simulink model "pipeline_12bit_not_ideal"  (R2017b)
settings: Solver=FixedStepAuto  StartTime=0.0  StopTime=5000*ts  FixedStep=ts  RelTol=1e-3
values from neighbouring files (symbols this model uses):
  bits_number = 12    [launch_pipeline_12ibt.m]
  fin = antismear(fin_pre,fs,nfft)    [launch_pipeline_12ibt.m]
  ts = 1/fs    (= 1)    [launch_pipeline_12ibt.m]
undefined symbols (not defined in the file or in its folder): clock
libraries: SDtoolbox x8
settings Model: Creator=umi  LastModifiedBy=SHUOGE
settings DataIOCC: LimitDataPoints=on  SaveFormat=Array  SaveOutput=off  SaveTime=off
settings OptimizationCC: ExpressionDepthLimit=2147483647  LifeSpan=inf
settings DebuggingCC: UnderspecifiedInitializationDetection=Classic  MergeDetectMultiDrivingBlocksExec=none  SolverPrmCheckMsg=warning  StateNameClashWarn=warning  SFUnexpectedBacktrackingDiag=warning  SFNoUnconditionalDefaultTransitionDiag=warning  SFExecutionAtInitializationDiag=none
settings HardwareCC: ProdBitPerPointer=32  ProdBitPerSizeT=32  ProdBitPerPtrDiffT=32  ProdLargestAtomicFloat=None  ProdIntDivRoundTo=Undefined  ProdEndianess=Unspecified  ProdWordSize=32  ProdHWDeviceType=32-bit Generic
settings ModelReferenceCC: PropagateSignalLabelsOutOfModel=off
settings CodeAppCC: StateflowObjectComments=on
settings GRTTargetCC: TargetLangStandard=C89/C90 (ANSI)  GeneratePreprocessorConditionals=Disable all  CombineOutputUpdateFcns=off  GRTInterface=on
settings ConfigComp: CovMetricSettings=dw  CovHtmlReporting=on  CovSaveCumulativeToWorkspaceVar=on  CovSaveSingleToWorkspaceVar=on  CovExternalEMLEnable=off  CovSFcnEnable=off

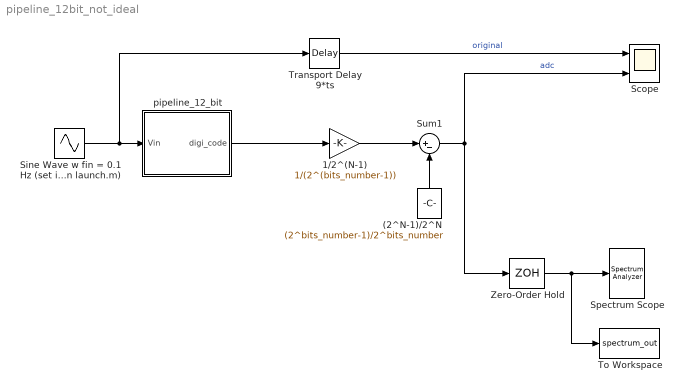
== system pipeline_12bit_not_ideal ==
  (2^N-1)/2^N : Constant  Value=(2^bits_number-1)/2^bits_number
  1/2^(N-1) : Gain  Gain=1/(2^(bits_number-1))
  Scope : Scope  NumInputPorts=2
  Sine Wave w fin = 0.1 Hz (set in launch.m) : Sin  Frequency=2*pi*fin  SampleTime=0
  Spectrum Scope : SpectrumAnalyzer
  Sum1 : Sum  Inputs=|+-
  To Workspace : ToWorkspace  VariableName=spectrum_out  SampleTime=-1
  Transport Delay 9*ts : TransportDelay  DelayTime=9
  Zero-Order Hold : ZeroOrderHold
  pipeline_12_bit : Subsystem
  wires:
  Sum1/1 -> Scope/2, Zero-Order Hold/1  "adc"
  (2^N-1)/2^N/1 -> Sum1/2
  1/2^(N-1)/1 -> Sum1/1
  pipeline_12_bit/1(digi_code) -> 1/2^(N-1)/1
  Sine Wave w fin = 0.1 Hz (set in launch.m)/1 -> pipeline_12_bit/1(Vin), Transport Delay 9*ts/1
  Zero-Order Hold/1 -> To Workspace/1, Spectrum Scope/1
  Transport Delay 9*ts/1 -> Scope/1  "original"

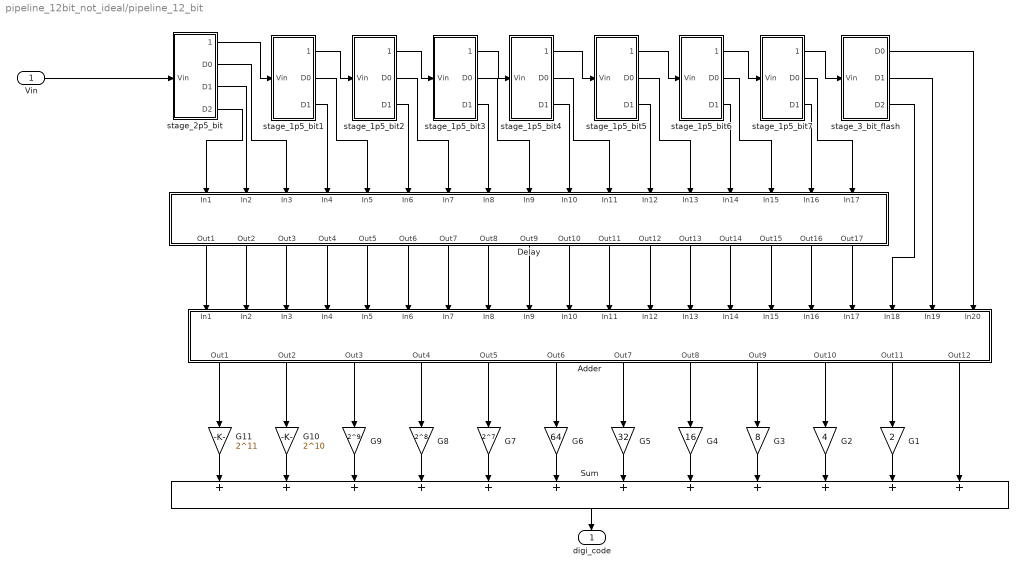
== system pipeline_12bit_not_ideal/pipeline_12_bit ==
  Vin : Inport
  Adder : Subsystem
  Delay : Subsystem
  G1 : Gain  Gain=2
  G10 : Gain  Gain=2^10
  G11 : Gain  Gain=2^11
  G2 : Gain  Gain=4
  G3 : Gain  Gain=8
  G4 : Gain  Gain=16
  G5 : Gain  Gain=32
  G6 : Gain  Gain=64
  G7 : Gain  Gain=2^7
  G8 : Gain  Gain=2^8
  G9 : Gain  Gain=2^9
  Sum : Sum  Inputs=++++++++++++
  stage_1p5_bit1 : Subsystem
  stage_1p5_bit2 : Subsystem
  stage_1p5_bit3 : Subsystem
  stage_1p5_bit4 : Subsystem
  stage_1p5_bit5 : Subsystem
  stage_1p5_bit6 : Subsystem
  stage_1p5_bit7 : Subsystem
  stage_2p5_bit : Subsystem
  stage_3_bit_flash : Subsystem
  digi_code : Outport
  wires:
  G1/1 -> Sum/11
  stage_2p5_bit/4(D2) -> Delay/1(In1)
  stage_2p5_bit/3(D1) -> Delay/2(In2)
  stage_2p5_bit/2(D0) -> Delay/3(In3)
  stage_1p5_bit1/3(D1) -> Delay/4(In4)
  stage_1p5_bit1/2(D0) -> Delay/5(In5)
  stage_1p5_bit2/3(D1) -> Delay/6(In6)
  stage_1p5_bit2/2(D0) -> Delay/7(In7)
  G2/1 -> Sum/10
  G3/1 -> Sum/9
  G4/1 -> Sum/8
  G5/1 -> Sum/7
  G6/1 -> Sum/6
  G7/1 -> Sum/5
  G8/1 -> Sum/4
  G9/1 -> Sum/3
  G10/1 -> Sum/2
  G11/1 -> Sum/1
  stage_3_bit_flash/3(D2) -> Adder/18(In18)
  stage_3_bit_flash/2(D1) -> Adder/19(In19)
  stage_3_bit_flash/1(D0) -> Adder/20(In20)
  Adder/1(Out1) -> G11/1
  Adder/2(Out2) -> G10/1
  Adder/3(Out3) -> G9/1
  Adder/4(Out4) -> G8/1
  Adder/5(Out5) -> G7/1
  Adder/12(Out12) -> Sum/12
  Adder/11(Out11) -> G1/1
  Adder/10(Out10) -> G2/1
  Adder/9(Out9) -> G3/1
  Adder/8(Out8) -> G4/1
  Adder/7(Out7) -> G5/1
  Adder/6(Out6) -> G6/1
  stage_1p5_bit1/1(Residue) -> stage_1p5_bit2/1(Vin)
  stage_1p5_bit2/1(Residue) -> stage_1p5_bit3/1(Vin)
  stage_1p5_bit3/1(Residue) -> stage_1p5_bit4/1(Vin)
  stage_1p5_bit4/1(Residue) -> stage_1p5_bit5/1(Vin)
  stage_2p5_bit/1(Residue) -> stage_1p5_bit1/1(Vin)
  stage_1p5_bit5/1(Residue) -> stage_1p5_bit6/1(Vin)
  stage_1p5_bit7/1(Residue) -> stage_3_bit_flash/1(Vin)
  stage_1p5_bit6/1(Residue) -> stage_1p5_bit7/1(Vin)
  Sum/1 -> digi_code/1
  stage_1p5_bit3/3(D1) -> Delay/8(In8)
  stage_1p5_bit3/2(D0) -> Delay/9(In9)
  stage_1p5_bit4/3(D1) -> Delay/10(In10)
  stage_1p5_bit4/2(D0) -> Delay/11(In11)
  stage_1p5_bit7/2(D0) -> Delay/17(In17)
  stage_1p5_bit7/3(D1) -> Delay/16(In16)
  stage_1p5_bit6/2(D0) -> Delay/15(In15)
  stage_1p5_bit6/3(D1) -> Delay/14(In14)
  stage_1p5_bit5/2(D0) -> Delay/13(In13)
  stage_1p5_bit5/3(D1) -> Delay/12(In12)
  Delay/1(Out1) -> Adder/1(In1)
  Delay/2(Out2) -> Adder/2(In2)
  Delay/3(Out3) -> Adder/3(In3)
  Delay/4(Out4) -> Adder/4(In4)
  Delay/5(Out5) -> Adder/5(In5)
  Delay/6(Out6) -> Adder/6(In6)
  Delay/7(Out7) -> Adder/7(In7)
  Delay/8(Out8) -> Adder/8(In8)
  Delay/9(Out9) -> Adder/9(In9)
  Delay/10(Out10) -> Adder/10(In10)
  Delay/12(Out12) -> Adder/12(In12)
  Delay/13(Out13) -> Adder/13(In13)
  Delay/14(Out14) -> Adder/14(In14)
  Delay/15(Out15) -> Adder/15(In15)
  Delay/16(Out16) -> Adder/16(In16)
  Delay/17(Out17) -> Adder/17(In17)
  Delay/11(Out11) -> Adder/11(In11)
  Vin/1 -> stage_2p5_bit/1(Vin)

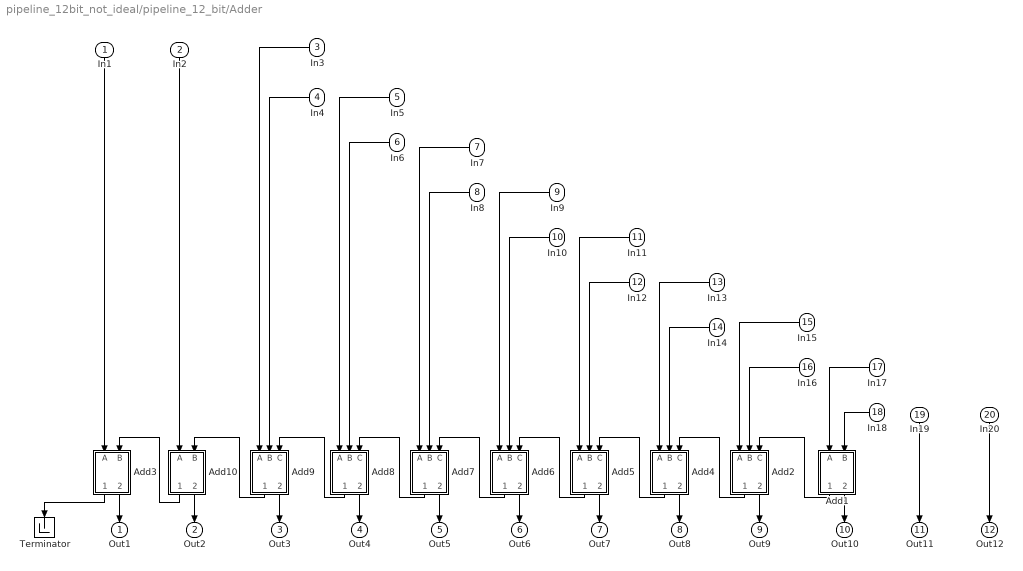
== system pipeline_12bit_not_ideal/pipeline_12_bit/Adder ==
  In1 : Inport
  In2 : Inport  Port=2
  In3 : Inport  Port=3
  In4 : Inport  Port=4
  In5 : Inport  Port=5
  In6 : Inport  Port=6
  In7 : Inport  Port=7
  In8 : Inport  Port=8
  In9 : Inport  Port=9
  In10 : Inport  Port=10
  In11 : Inport  Port=11
  In12 : Inport  Port=12
  In13 : Inport  Port=13
  In14 : Inport  Port=14
  In15 : Inport  Port=15
  In16 : Inport  Port=16
  In17 : Inport  Port=17
  In18 : Inport  Port=18
  In19 : Inport  Port=19
  In20 : Inport  Port=20
  Add1 : Subsystem
  Add10 : Subsystem
  Add2 : Subsystem
  Add3 : Subsystem
  Add4 : Subsystem
  Add5 : Subsystem
  Add6 : Subsystem
  Add7 : Subsystem
  Add8 : Subsystem
  Add9 : Subsystem
  Terminator : Terminator
  Out1 : Outport
  Out2 : Outport  Port=2
  Out3 : Outport  Port=3
  Out4 : Outport  Port=4
  Out5 : Outport  Port=5
  Out6 : Outport  Port=6
  Out7 : Outport  Port=7
  Out8 : Outport  Port=8
  Out9 : Outport  Port=9
  Out10 : Outport  Port=10
  Out11 : Outport  Port=11
  Out12 : Outport  Port=12
  wires:
  In20/1 -> Out12/1
  In19/1 -> Out11/1
  In18/1 -> Add1/2(B)
  In17/1 -> Add1/1(A)
  Add1/2(Sum) -> Out10/1
  Add1/1(Carry) -> Add2/3(C)
  Add2/2(Sum) -> Out9/1
  In14/1 -> Add4/2(B)
  In13/1 -> Add4/1(A)
  Add5/2(Sum) -> Out7/1
  Add4/1(Carry) -> Add5/3(C)
  In12/1 -> Add5/2(B)
  In11/1 -> Add5/1(A)
  Add6/2(Sum) -> Out6/1
  Add5/1(Carry) -> Add6/3(C)
  In10/1 -> Add6/2(B)
  In9/1 -> Add6/1(A)
  Add7/2(Sum) -> Out5/1
  Add6/1(Carry) -> Add7/3(C)
  In8/1 -> Add7/2(B)
  In7/1 -> Add7/1(A)
  Add8/2(Sum) -> Out4/1
  Add7/1(Carry) -> Add8/3(C)
  In6/1 -> Add8/2(B)
  In5/1 -> Add8/1(A)
  Add8/1(Carry) -> Add9/3(C)
  Add9/2(Sum) -> Out3/1
  In4/1 -> Add9/2(B)
  In3/1 -> Add9/1(A)
  Add10/2(Sum) -> Out2/1
  Add9/1(Carry) -> Add10/2(B)
  In2/1 -> Add10/1(A)
  In16/1 -> Add2/2(B)
  In15/1 -> Add2/1(A)
  Add2/1(Carry) -> Add4/3(C)
  Add4/2(Sum) -> Out8/1
  Add10/1(Carry) -> Add3/2(B)
  Add3/2(Sum) -> Out1/1
  In1/1 -> Add3/1(A)
  Add3/1(Carry) -> Terminator/1

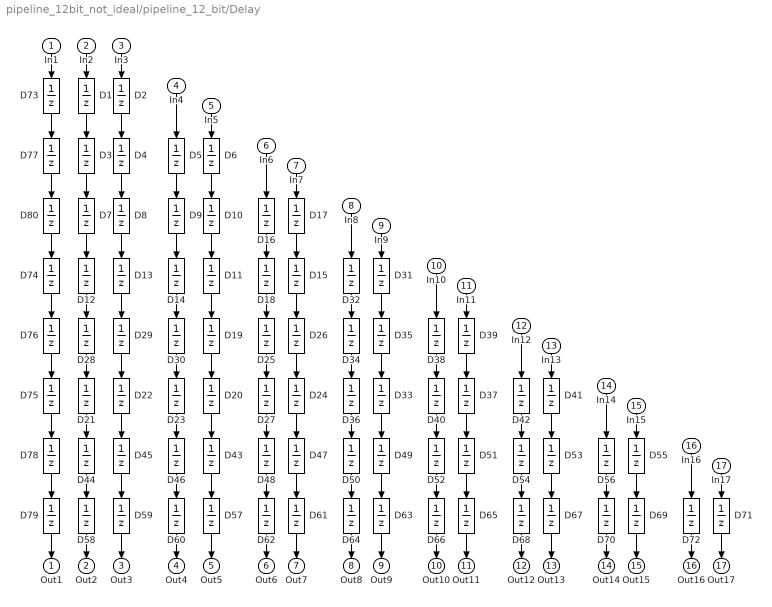
== system pipeline_12bit_not_ideal/pipeline_12_bit/Delay ==
  In1 : Inport
  In2 : Inport  Port=2
  In3 : Inport  Port=3
  In4 : Inport  Port=4
  In5 : Inport  Port=5
  In6 : Inport  Port=6
  In7 : Inport  Port=7
  In8 : Inport  Port=8
  In9 : Inport  Port=9
  In10 : Inport  Port=10
  In11 : Inport  Port=11
  In12 : Inport  Port=12
  In13 : Inport  Port=13
  In14 : Inport  Port=14
  In15 : Inport  Port=15
  In16 : Inport  Port=16
  In17 : Inport  Port=17
  D{1..80} (80 alike) : UnitDelay  SampleTime=-1
  Out1 : Outport
  Out2 : Outport  Port=2
  Out3 : Outport  Port=3
  Out4 : Outport  Port=4
  Out5 : Outport  Port=5
  Out6 : Outport  Port=6
  Out7 : Outport  Port=7
  Out8 : Outport  Port=8
  Out9 : Outport  Port=9
  Out10 : Outport  Port=10
  Out11 : Outport  Port=11
  Out12 : Outport  Port=12
  Out13 : Outport  Port=13
  Out14 : Outport  Port=14
  Out15 : Outport  Port=15
  Out16 : Outport  Port=16
  Out17 : Outport  Port=17
  wires:
  D2/1 -> D4/1
  D1/1 -> D3/1
  In2/1 -> D1/1
  In3/1 -> D2/1
  In5/1 -> D6/1
  In4/1 -> D5/1
  D4/1 -> D8/1
  D3/1 -> D7/1
  D6/1 -> D10/1
  D5/1 -> D9/1
  D8/1 -> D13/1
  D7/1 -> D12/1
  D10/1 -> D11/1
  D9/1 -> D14/1
  In7/1 -> D17/1
  In6/1 -> D16/1
  D17/1 -> D15/1
  D16/1 -> D18/1
  D15/1 -> D26/1
  D18/1 -> D25/1
  D13/1 -> D29/1
  D12/1 -> D28/1
  D11/1 -> D19/1
  D14/1 -> D30/1
  D29/1 -> D22/1
  D28/1 -> D21/1
  D19/1 -> D20/1
  D30/1 -> D23/1
  D26/1 -> D24/1
  D25/1 -> D27/1
  D24/1 -> D47/1
  D27/1 -> D48/1
  D31/1 -> D35/1
  D32/1 -> D34/1
  D35/1 -> D33/1
  D34/1 -> D36/1
  D33/1 -> D49/1
  D36/1 -> D50/1
  D39/1 -> D37/1
  D38/1 -> D40/1
  D37/1 -> D51/1
  D40/1 -> D52/1
  D41/1 -> D53/1
  D42/1 -> D54/1
  D47/1 -> D61/1
  D49/1 -> D63/1
  D50/1 -> D64/1
  D51/1 -> D65/1
  D52/1 -> D66/1
  D53/1 -> D67/1
  D54/1 -> D68/1
  D21/1 -> D44/1
  D22/1 -> D45/1
  D23/1 -> D46/1
  D20/1 -> D43/1
  In15/1 -> D55/1
  In14/1 -> D56/1
  D55/1 -> D69/1
  D56/1 -> D70/1
  D61/1 -> Out7/1
  D62/1 -> Out6/1
  D63/1 -> Out9/1
  D64/1 -> Out8/1
  D65/1 -> Out11/1
  D66/1 -> Out10/1
  D67/1 -> Out13/1
  D68/1 -> Out12/1
  D44/1 -> D58/1
  D45/1 -> D59/1
  D46/1 -> D60/1
  D43/1 -> D57/1
  D69/1 -> Out15/1
  D70/1 -> Out14/1
  D48/1 -> D62/1
  D71/1 -> Out17/1
  D72/1 -> Out16/1
  D73/1 -> D77/1
  D77/1 -> D80/1
  D80/1 -> D74/1
  D74/1 -> D76/1
  D76/1 -> D75/1
  D75/1 -> D78/1
  D78/1 -> D79/1
  In1/1 -> D73/1
  In8/1 -> D32/1
  In17/1 -> D71/1
  In16/1 -> D72/1
  In13/1 -> D41/1
  In12/1 -> D42/1
  In11/1 -> D39/1
  In10/1 -> D38/1
  In9/1 -> D31/1
  D79/1 -> Out1/1
  D58/1 -> Out2/1
  D59/1 -> Out3/1
  D60/1 -> Out4/1
  D57/1 -> Out5/1

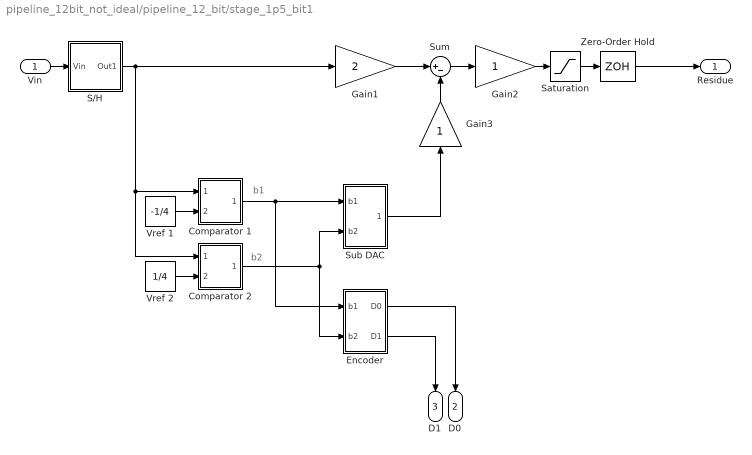
== system pipeline_12bit_not_ideal/pipeline_12_bit/stage_1p5_bit1 ==
  note: b2
  note: b1
  Vin : Inport
  Comparator 1 : Subsystem
  Comparator 2 : Subsystem
  Encoder : Subsystem
  Gain1 : Gain  Gain=2
  Gain2 : Gain
  Gain3 : Gain
  S/H : Subsystem
  Saturation : Saturate  UpperLimit=1  LowerLimit=-1
  Sub DAC : Subsystem
  Sum : Sum  Inputs=|+-
  Vref 1 : Constant  Value=-1/4
  Vref 2 : Constant  Value=1/4
  Zero-Order Hold : ZeroOrderHold  SampleTime=ts
  Residue : Outport
  D0 : Outport  Port=2
  D1 : Outport  Port=3
  wires:
  Vref 1/1 -> Comparator 1/2(Vref)
  Gain1/1 -> Sum/1
  Gain3/1 -> Sum/2
  Sum/1 -> Gain2/1
  Saturation/1 -> Zero-Order Hold/1
  Zero-Order Hold/1 -> Residue/1
  Gain2/1 -> Saturation/1
  Vref 2/1 -> Comparator 2/2(Vref)
  Comparator 2/1(Out) -> Sub DAC/2(b2), Encoder/2(b2)
  Vin/1 -> S/H/1(Vin)
  Comparator 1/1(Out) -> Encoder/1(b1), Sub DAC/1(b1)
  S/H/1(Out1) -> Comparator 1/1(Vin), Comparator 2/1(Vin), Gain1/1
  Sub DAC/1(Vdac) -> Gain3/1
  Encoder/1(D0) -> D0/1
  Encoder/2(D1) -> D1/1

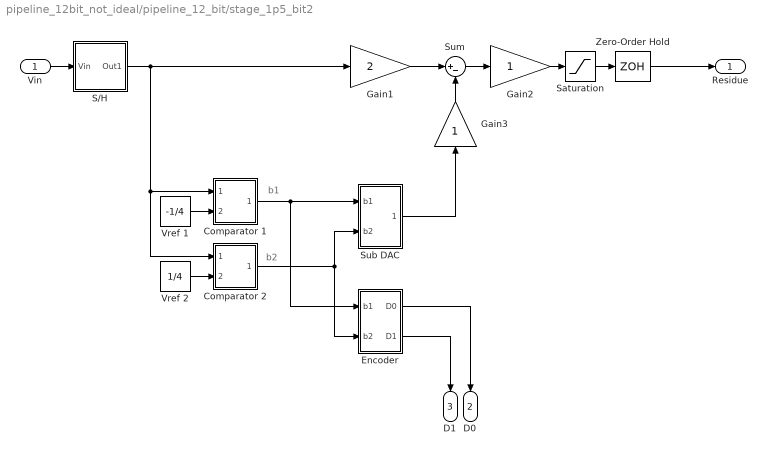
== system pipeline_12bit_not_ideal/pipeline_12_bit/stage_1p5_bit2 ==
  note: b2
  note: b1
  Vin : Inport
  Comparator 1 : Subsystem
  Comparator 2 : Subsystem
  Encoder : Subsystem
  Gain1 : Gain  Gain=2
  Gain2 : Gain
  Gain3 : Gain
  S/H : Subsystem
  Saturation : Saturate  UpperLimit=1  LowerLimit=-1
  Sub DAC : Subsystem
  Sum : Sum  Inputs=|+-
  Vref 1 : Constant  Value=-1/4
  Vref 2 : Constant  Value=1/4
  Zero-Order Hold : ZeroOrderHold  SampleTime=ts
  Residue : Outport
  D0 : Outport  Port=2
  D1 : Outport  Port=3
  wires:
  Vref 1/1 -> Comparator 1/2(Vref)
  Gain1/1 -> Sum/1
  Gain3/1 -> Sum/2
  Sum/1 -> Gain2/1
  Saturation/1 -> Zero-Order Hold/1
  Zero-Order Hold/1 -> Residue/1
  Gain2/1 -> Saturation/1
  Vref 2/1 -> Comparator 2/2(Vref)
  Comparator 2/1(Out) -> Sub DAC/2(b2), Encoder/2(b2)
  Vin/1 -> S/H/1(Vin)
  Comparator 1/1(Out) -> Encoder/1(b1), Sub DAC/1(b1)
  S/H/1(Out1) -> Comparator 1/1(Vin), Comparator 2/1(Vin), Gain1/1
  Sub DAC/1(Vdac) -> Gain3/1
  Encoder/1(D0) -> D0/1
  Encoder/2(D1) -> D1/1

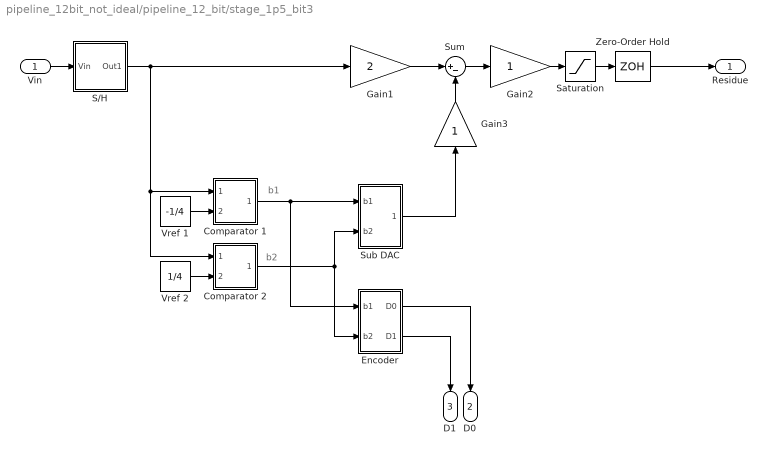
== system pipeline_12bit_not_ideal/pipeline_12_bit/stage_1p5_bit3 ==
  note: b2
  note: b1
  Vin : Inport
  Comparator 1 : Subsystem
  Comparator 2 : Subsystem
  Encoder : Subsystem
  Gain1 : Gain  Gain=2
  Gain2 : Gain
  Gain3 : Gain
  S/H : Subsystem
  Saturation : Saturate  UpperLimit=1  LowerLimit=-1
  Sub DAC : Subsystem
  Sum : Sum  Inputs=|+-
  Vref 1 : Constant  Value=-1/4
  Vref 2 : Constant  Value=1/4
  Zero-Order Hold : ZeroOrderHold  SampleTime=ts
  Residue : Outport
  D0 : Outport  Port=2
  D1 : Outport  Port=3
  wires:
  Vref 1/1 -> Comparator 1/2(Vref)
  Gain1/1 -> Sum/1
  Gain3/1 -> Sum/2
  Sum/1 -> Gain2/1
  Saturation/1 -> Zero-Order Hold/1
  Zero-Order Hold/1 -> Residue/1
  Gain2/1 -> Saturation/1
  Vref 2/1 -> Comparator 2/2(Vref)
  Comparator 2/1(Out) -> Sub DAC/2(b2), Encoder/2(b2)
  Vin/1 -> S/H/1(Vin)
  Comparator 1/1(Out) -> Encoder/1(b1), Sub DAC/1(b1)
  S/H/1(Out1) -> Comparator 1/1(Vin), Comparator 2/1(Vin), Gain1/1
  Sub DAC/1(Vdac) -> Gain3/1
  Encoder/1(D0) -> D0/1
  Encoder/2(D1) -> D1/1

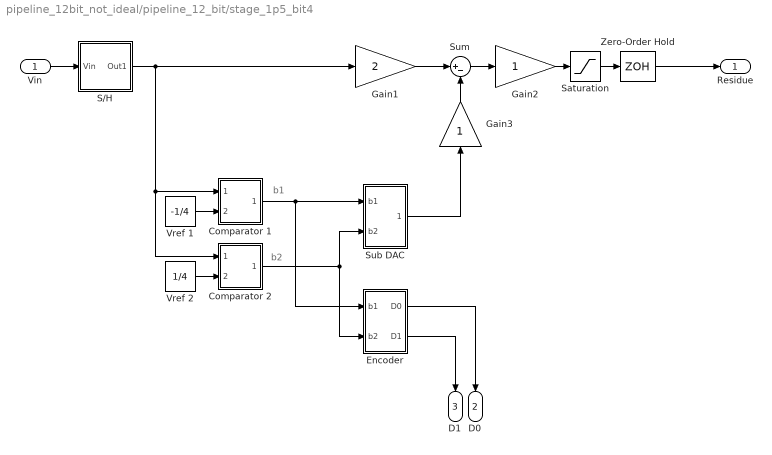
== system pipeline_12bit_not_ideal/pipeline_12_bit/stage_1p5_bit4 ==
  note: b2
  note: b1
  Vin : Inport
  Comparator 1 : Subsystem
  Comparator 2 : Subsystem
  Encoder : Subsystem
  Gain1 : Gain  Gain=2
  Gain2 : Gain
  Gain3 : Gain
  S/H : Subsystem
  Saturation : Saturate  UpperLimit=1  LowerLimit=-1
  Sub DAC : Subsystem
  Sum : Sum  Inputs=|+-
  Vref 1 : Constant  Value=-1/4
  Vref 2 : Constant  Value=1/4
  Zero-Order Hold : ZeroOrderHold  SampleTime=ts
  Residue : Outport
  D0 : Outport  Port=2
  D1 : Outport  Port=3
  wires:
  Vref 1/1 -> Comparator 1/2(Vref)
  Gain1/1 -> Sum/1
  Gain3/1 -> Sum/2
  Sum/1 -> Gain2/1
  Saturation/1 -> Zero-Order Hold/1
  Zero-Order Hold/1 -> Residue/1
  Gain2/1 -> Saturation/1
  Vref 2/1 -> Comparator 2/2(Vref)
  Comparator 2/1(Out) -> Sub DAC/2(b2), Encoder/2(b2)
  Vin/1 -> S/H/1(Vin)
  Comparator 1/1(Out) -> Encoder/1(b1), Sub DAC/1(b1)
  S/H/1(Out1) -> Comparator 1/1(Vin), Comparator 2/1(Vin), Gain1/1
  Sub DAC/1(Vdac) -> Gain3/1
  Encoder/1(D0) -> D0/1
  Encoder/2(D1) -> D1/1

== system pipeline_12bit_not_ideal/pipeline_12_bit/stage_1p5_bit5 ==
  note: b2
  note: b1
  Vin : Inport
  Comparator 1 : Subsystem
  Comparator 2 : Subsystem
  Encoder : Subsystem
  Gain1 : Gain  Gain=2
  Gain2 : Gain
  Gain3 : Gain
  S/H : Subsystem
  Saturation : Saturate  UpperLimit=1  LowerLimit=-1
  Sub DAC : Subsystem
  Sum : Sum  Inputs=|+-
  Vref 1 : Constant  Value=-1/4
  Vref 2 : Constant  Value=1/4
  Zero-Order Hold : ZeroOrderHold  SampleTime=ts
  Residue : Outport
  D0 : Outport  Port=2
  D1 : Outport  Port=3
  wires:
  Vref 1/1 -> Comparator 1/2(Vref)
  Gain1/1 -> Sum/1
  Gain3/1 -> Sum/2
  Sum/1 -> Gain2/1
  Saturation/1 -> Zero-Order Hold/1
  Zero-Order Hold/1 -> Residue/1
  Gain2/1 -> Saturation/1
  Vref 2/1 -> Comparator 2/2(Vref)
  Comparator 2/1(Out) -> Sub DAC/2(b2), Encoder/2(b2)
  Vin/1 -> S/H/1(Vin)
  Comparator 1/1(Out) -> Encoder/1(b1), Sub DAC/1(b1)
  S/H/1(Out1) -> Comparator 1/1(Vin), Comparator 2/1(Vin), Gain1/1
  Sub DAC/1(Vdac) -> Gain3/1
  Encoder/1(D0) -> D0/1
  Encoder/2(D1) -> D1/1

== system pipeline_12bit_not_ideal/pipeline_12_bit/stage_1p5_bit6 ==
  note: b2
  note: b1
  Vin : Inport
  Comparator 1 : Subsystem
  Comparator 2 : Subsystem
  Encoder : Subsystem
  Gain1 : Gain  Gain=2
  Gain2 : Gain
  Gain3 : Gain
  S/H : Subsystem
  Saturation : Saturate  UpperLimit=1  LowerLimit=-1
  Sub DAC : Subsystem
  Sum : Sum  Inputs=|+-
  Vref 1 : Constant  Value=-1/4
  Vref 2 : Constant  Value=1/4
  Zero-Order Hold : ZeroOrderHold  SampleTime=ts
  Residue : Outport
  D0 : Outport  Port=2
  D1 : Outport  Port=3
  wires:
  Vref 1/1 -> Comparator 1/2(Vref)
  Gain1/1 -> Sum/1
  Gain3/1 -> Sum/2
  Sum/1 -> Gain2/1
  Saturation/1 -> Zero-Order Hold/1
  Zero-Order Hold/1 -> Residue/1
  Gain2/1 -> Saturation/1
  Vref 2/1 -> Comparator 2/2(Vref)
  Comparator 2/1(Out) -> Sub DAC/2(b2), Encoder/2(b2)
  Vin/1 -> S/H/1(Vin)
  Comparator 1/1(Out) -> Encoder/1(b1), Sub DAC/1(b1)
  S/H/1(Out1) -> Comparator 1/1(Vin), Comparator 2/1(Vin), Gain1/1
  Sub DAC/1(Vdac) -> Gain3/1
  Encoder/1(D0) -> D0/1
  Encoder/2(D1) -> D1/1

== system pipeline_12bit_not_ideal/pipeline_12_bit/stage_1p5_bit7 ==
  note: b2
  note: b1
  Vin : Inport
  Comparator 1 : Subsystem
  Comparator 2 : Subsystem
  Encoder : Subsystem
  Gain1 : Gain  Gain=2
  Gain2 : Gain
  Gain3 : Gain
  S/H : Subsystem
  Saturation : Saturate  UpperLimit=1  LowerLimit=-1
  Sub DAC : Subsystem
  Sum : Sum  Inputs=|+-
  Vref 1 : Constant  Value=-1/4
  Vref 2 : Constant  Value=1/4
  Zero-Order Hold : ZeroOrderHold  SampleTime=ts
  Residue : Outport
  D0 : Outport  Port=2
  D1 : Outport  Port=3
  wires:
  Vref 1/1 -> Comparator 1/2(Vref)
  Gain1/1 -> Sum/1
  Gain3/1 -> Sum/2
  Sum/1 -> Gain2/1
  Saturation/1 -> Zero-Order Hold/1
  Zero-Order Hold/1 -> Residue/1
  Gain2/1 -> Saturation/1
  Vref 2/1 -> Comparator 2/2(Vref)
  Comparator 2/1(Out) -> Sub DAC/2(b2), Encoder/2(b2)
  Vin/1 -> S/H/1(Vin)
  Comparator 1/1(Out) -> Encoder/1(b1), Sub DAC/1(b1)
  S/H/1(Out1) -> Comparator 1/1(Vin), Comparator 2/1(Vin), Gain1/1
  Sub DAC/1(Vdac) -> Gain3/1
  Encoder/1(D0) -> D0/1
  Encoder/2(D1) -> D1/1

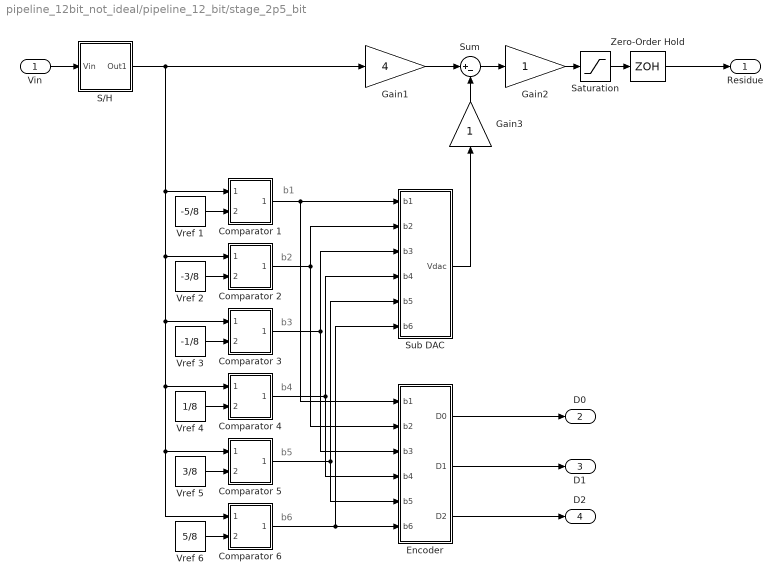
== system pipeline_12bit_not_ideal/pipeline_12_bit/stage_2p5_bit ==
  note: b2
  note: b1
  note: b3
  note: b4
  note: b5
  note: b6
  Vin : Inport
  Comparator 1 : Subsystem
  Comparator 2 : Subsystem
  Comparator 3 : Subsystem
  Comparator 4 : Subsystem
  Comparator 5 : Subsystem
  Comparator 6 : Subsystem
  Encoder : Subsystem
  Gain1 : Gain  Gain=4
  Gain2 : Gain
  Gain3 : Gain
  S/H : Subsystem
  Saturation : Saturate  UpperLimit=1  LowerLimit=-1
  Sub DAC : Subsystem
  Sum : Sum  Inputs=|+-
  Vref 1 : Constant  Value=-5/8
  Vref 2 : Constant  Value=-3/8
  Vref 3 : Constant  Value=-1/8
  Vref 4 : Constant  Value=1/8
  Vref 5 : Constant  Value=3/8
  Vref 6 : Constant  Value=5/8
  Zero-Order Hold : ZeroOrderHold  SampleTime=ts
  Residue : Outport
  D0 : Outport  Port=2
  D1 : Outport  Port=3
  D2 : Outport  Port=4
  wires:
  Vref 1/1 -> Comparator 1/2(Vref)
  Sub DAC/1(Vdac) -> Gain3/1
  Gain1/1 -> Sum/1
  Gain3/1 -> Sum/2
  Sum/1 -> Gain2/1
  Saturation/1 -> Zero-Order Hold/1
  Zero-Order Hold/1 -> Residue/1
  Gain2/1 -> Saturation/1
  Vref 2/1 -> Comparator 2/2(Vref)
  Vin/1 -> S/H/1(Vin)
  Comparator 1/1(Out) -> Sub DAC/1(b1), Encoder/1(b1)
  Vref 3/1 -> Comparator 3/2(Vref)
  Vref 4/1 -> Comparator 4/2(Vref)
  Vref 5/1 -> Comparator 5/2(Vref)
  Vref 6/1 -> Comparator 6/2(Vref)
  Comparator 2/1(Out) -> Sub DAC/2(b2), Encoder/2(b2)
  Comparator 3/1(Out) -> Sub DAC/3(b3), Encoder/3(b3)
  Comparator 4/1(Out) -> Sub DAC/4(b4), Encoder/4(b4)
  Comparator 5/1(Out) -> Sub DAC/5(b5), Encoder/5(b5)
  Comparator 6/1(Out) -> Sub DAC/6(b6), Encoder/6(b6)
  Encoder/1(D0) -> D0/1
  Encoder/3(D2) -> D2/1
  Encoder/2(D1) -> D1/1
  S/H/1(Out1) -> Comparator 1/1(Vin), Comparator 2/1(Vin), Comparator 3/1(Vin), Comparator 4/1(Vin), Comparator 6/1(Vin), Comparator 5/1(Vin), Gain1/1

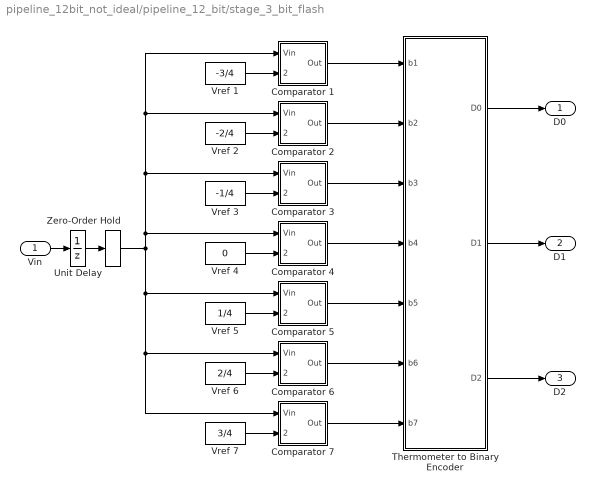
== system pipeline_12bit_not_ideal/pipeline_12_bit/stage_3_bit_flash ==
  Vin : Inport
  Comparator 1 : Subsystem
  Comparator 2 : Subsystem
  Comparator 3 : Subsystem
  Comparator 4 : Subsystem
  Comparator 5 : Subsystem
  Comparator 6 : Subsystem
  Comparator 7 : Subsystem
  Thermometer to Binary Encoder : Subsystem
  Unit Delay : UnitDelay  SampleTime=-1
  Vref 1 : Constant  Value=-3/4
  Vref 2 : Constant  Value=-2/4
  Vref 3 : Constant  Value=-1/4
  Vref 4 : Constant  Value=0
  Vref 5 : Constant  Value=1/4
  Vref 6 : Constant  Value=2/4
  Vref 7 : Constant  Value=3/4
  Zero-Order Hold : ZeroOrderHold  SampleTime=ts
  D0 : Outport
  D1 : Outport  Port=2
  D2 : Outport  Port=3
  wires:
  Vin/1 -> Unit Delay/1
  Vref 1/1 -> Comparator 1/2(Vref)
  Thermometer to Binary Encoder/1(D0) -> D0/1
  Thermometer to Binary Encoder/2(D1) -> D1/1
  Thermometer to Binary Encoder/3(D2) -> D2/1
  Comparator 1/1(Out) -> Thermometer to Binary Encoder/1(b1)
  Vref 2/1 -> Comparator 2/2(Vref)
  Comparator 2/1(Out) -> Thermometer to Binary Encoder/2(b2)
  Vref 3/1 -> Comparator 3/2(Vref)
  Comparator 3/1(Out) -> Thermometer to Binary Encoder/3(b3)
  Vref 4/1 -> Comparator 4/2(Vref)
  Comparator 4/1(Out) -> Thermometer to Binary Encoder/4(b4)
  Vref 5/1 -> Comparator 5/2(Vref)
  Comparator 5/1(Out) -> Thermometer to Binary Encoder/5(b5)
  Vref 6/1 -> Comparator 6/2(Vref)
  Comparator 6/1(Out) -> Thermometer to Binary Encoder/6(b6)
  Vref 7/1 -> Comparator 7/2(Vref)
  Comparator 7/1(Out) -> Thermometer to Binary Encoder/7(b7)
  Zero-Order Hold/1 -> Comparator 1/1(Vin), Comparator 2/1(Vin), Comparator 3/1(Vin), Comparator 4/1(Vin), Comparator 5/1(Vin), Comparator 6/1(Vin), Comparator 7/1(Vin)
  Unit Delay/1 -> Zero-Order Hold/1

== system pipeline_12bit_not_ideal/pipeline_12_bit/Adder/Add1 ==
  A : Inport
  B : Inport  Port=2
  Combinatorial Logic1 : CombinatorialLogic  TruthTable=[0 0;1 0 ;1 0;0 1;1 0;0 1;0 1;1 1]
  Constant : Constant  Value=0
  Data Type Conversion : DataTypeConversion  OutDataTypeStr=boolean
  Data Type Conversion1 : DataTypeConversion  OutDataTypeStr=double
  Demux : Demux  Outputs=2
  Mux : Mux  Inputs=3
  Carry : Outport
  Sum : Outport  Port=2
  wires:
  Demux/1 -> Sum/1
  Demux/2 -> Carry/1
  Combinatorial Logic1/1 -> Data Type Conversion1/1
  Mux/1 -> Data Type Conversion/1
  A/1 -> Mux/3
  B/1 -> Mux/2
  Constant/1 -> Mux/1
  Data Type Conversion1/1 -> Demux/1
  Data Type Conversion/1 -> Combinatorial Logic1/1

== system pipeline_12bit_not_ideal/pipeline_12_bit/Adder/Add10 ==
  A : Inport
  B : Inport  Port=2
  Combinatorial Logic1 : CombinatorialLogic  TruthTable=[0 0;1 0 ;1 0;0 1;1 0;0 1;0 1;1 1]
  Constant : Constant  Value=0
  Data Type Conversion : DataTypeConversion  OutDataTypeStr=boolean
  Data Type Conversion1 : DataTypeConversion  OutDataTypeStr=double
  Demux : Demux  Outputs=2
  Mux : Mux  Inputs=3
  Carry : Outport
  Sum : Outport  Port=2
  wires:
  Demux/1 -> Sum/1
  Demux/2 -> Carry/1
  Combinatorial Logic1/1 -> Data Type Conversion1/1
  Mux/1 -> Data Type Conversion/1
  A/1 -> Mux/3
  B/1 -> Mux/2
  Constant/1 -> Mux/1
  Data Type Conversion1/1 -> Demux/1
  Data Type Conversion/1 -> Combinatorial Logic1/1

== system pipeline_12bit_not_ideal/pipeline_12_bit/Adder/Add2 ==
  A : Inport
  B : Inport  Port=2
  C : Inport  Port=3
  Combinatorial Logic1 : CombinatorialLogic  TruthTable=[0 0;1 0 ;1 0;0 1;1 0;0 1;0 1;1 1]
  Data Type Conversion : DataTypeConversion  OutDataTypeStr=boolean
  Data Type Conversion1 : DataTypeConversion  OutDataTypeStr=double
  Demux : Demux  Outputs=2
  Mux : Mux  Inputs=3
  Carry : Outport
  Sum : Outport  Port=2
  wires:
  Demux/1 -> Sum/1
  Demux/2 -> Carry/1
  Combinatorial Logic1/1 -> Data Type Conversion1/1
  Mux/1 -> Data Type Conversion/1
  A/1 -> Mux/3
  B/1 -> Mux/2
  C/1 -> Mux/1
  Data Type Conversion1/1 -> Demux/1
  Data Type Conversion/1 -> Combinatorial Logic1/1

== system pipeline_12bit_not_ideal/pipeline_12_bit/Adder/Add3 ==
  A : Inport
  B : Inport  Port=2
  Combinatorial Logic1 : CombinatorialLogic  TruthTable=[0 0;1 0 ;1 0;0 1;1 0;0 1;0 1;1 1]
  Constant : Constant  Value=0
  Data Type Conversion : DataTypeConversion  OutDataTypeStr=boolean
  Data Type Conversion1 : DataTypeConversion  OutDataTypeStr=double
  Demux : Demux  Outputs=2
  Mux : Mux  Inputs=3
  Carry : Outport
  Sum : Outport  Port=2
  wires:
  Demux/1 -> Sum/1
  Demux/2 -> Carry/1
  Combinatorial Logic1/1 -> Data Type Conversion1/1
  Mux/1 -> Data Type Conversion/1
  A/1 -> Mux/3
  B/1 -> Mux/2
  Constant/1 -> Mux/1
  Data Type Conversion1/1 -> Demux/1
  Data Type Conversion/1 -> Combinatorial Logic1/1

== system pipeline_12bit_not_ideal/pipeline_12_bit/Adder/Add4 ==
  A : Inport
  B : Inport  Port=2
  C : Inport  Port=3
  Combinatorial Logic1 : CombinatorialLogic  TruthTable=[0 0;1 0 ;1 0;0 1;1 0;0 1;0 1;1 1]
  Data Type Conversion : DataTypeConversion  OutDataTypeStr=boolean
  Data Type Conversion1 : DataTypeConversion  OutDataTypeStr=double
  Demux : Demux  Outputs=2
  Mux : Mux  Inputs=3
  Carry : Outport
  Sum : Outport  Port=2
  wires:
  Demux/1 -> Sum/1
  Demux/2 -> Carry/1
  Combinatorial Logic1/1 -> Data Type Conversion1/1
  Mux/1 -> Data Type Conversion/1
  A/1 -> Mux/3
  B/1 -> Mux/2
  C/1 -> Mux/1
  Data Type Conversion1/1 -> Demux/1
  Data Type Conversion/1 -> Combinatorial Logic1/1

== system pipeline_12bit_not_ideal/pipeline_12_bit/Adder/Add5 ==
  A : Inport
  B : Inport  Port=2
  C : Inport  Port=3
  Combinatorial Logic1 : CombinatorialLogic  TruthTable=[0 0;1 0 ;1 0;0 1;1 0;0 1;0 1;1 1]
  Data Type Conversion : DataTypeConversion  OutDataTypeStr=boolean
  Data Type Conversion1 : DataTypeConversion  OutDataTypeStr=double
  Demux : Demux  Outputs=2
  Mux : Mux  Inputs=3
  Carry : Outport
  Sum : Outport  Port=2
  wires:
  Demux/1 -> Sum/1
  Demux/2 -> Carry/1
  Combinatorial Logic1/1 -> Data Type Conversion1/1
  Mux/1 -> Data Type Conversion/1
  A/1 -> Mux/3
  B/1 -> Mux/2
  C/1 -> Mux/1
  Data Type Conversion1/1 -> Demux/1
  Data Type Conversion/1 -> Combinatorial Logic1/1

== system pipeline_12bit_not_ideal/pipeline_12_bit/Adder/Add6 ==
  A : Inport
  B : Inport  Port=2
  C : Inport  Port=3
  Combinatorial Logic1 : CombinatorialLogic  TruthTable=[0 0;1 0 ;1 0;0 1;1 0;0 1;0 1;1 1]
  Data Type Conversion : DataTypeConversion  OutDataTypeStr=boolean
  Data Type Conversion1 : DataTypeConversion  OutDataTypeStr=double
  Demux : Demux  Outputs=2
  Mux : Mux  Inputs=3
  Carry : Outport
  Sum : Outport  Port=2
  wires:
  Demux/1 -> Sum/1
  Demux/2 -> Carry/1
  Combinatorial Logic1/1 -> Data Type Conversion1/1
  Mux/1 -> Data Type Conversion/1
  A/1 -> Mux/3
  B/1 -> Mux/2
  C/1 -> Mux/1
  Data Type Conversion1/1 -> Demux/1
  Data Type Conversion/1 -> Combinatorial Logic1/1

== system pipeline_12bit_not_ideal/pipeline_12_bit/Adder/Add7 ==
  A : Inport
  B : Inport  Port=2
  C : Inport  Port=3
  Combinatorial Logic1 : CombinatorialLogic  TruthTable=[0 0;1 0 ;1 0;0 1;1 0;0 1;0 1;1 1]
  Data Type Conversion : DataTypeConversion  OutDataTypeStr=boolean
  Data Type Conversion1 : DataTypeConversion  OutDataTypeStr=double
  Demux : Demux  Outputs=2
  Mux : Mux  Inputs=3
  Carry : Outport
  Sum : Outport  Port=2
  wires:
  Demux/1 -> Sum/1
  Demux/2 -> Carry/1
  Combinatorial Logic1/1 -> Data Type Conversion1/1
  Mux/1 -> Data Type Conversion/1
  A/1 -> Mux/3
  B/1 -> Mux/2
  C/1 -> Mux/1
  Data Type Conversion1/1 -> Demux/1
  Data Type Conversion/1 -> Combinatorial Logic1/1

== system pipeline_12bit_not_ideal/pipeline_12_bit/Adder/Add8 ==
  A : Inport
  B : Inport  Port=2
  C : Inport  Port=3
  Combinatorial Logic1 : CombinatorialLogic  TruthTable=[0 0;1 0 ;1 0;0 1;1 0;0 1;0 1;1 1]
  Data Type Conversion : DataTypeConversion  OutDataTypeStr=boolean
  Data Type Conversion1 : DataTypeConversion  OutDataTypeStr=double
  Demux : Demux  Outputs=2
  Mux : Mux  Inputs=3
  Carry : Outport
  Sum : Outport  Port=2
  wires:
  Demux/1 -> Sum/1
  Demux/2 -> Carry/1
  Combinatorial Logic1/1 -> Data Type Conversion1/1
  Mux/1 -> Data Type Conversion/1
  A/1 -> Mux/3
  B/1 -> Mux/2
  C/1 -> Mux/1
  Data Type Conversion1/1 -> Demux/1
  Data Type Conversion/1 -> Combinatorial Logic1/1

== system pipeline_12bit_not_ideal/pipeline_12_bit/Adder/Add9 ==
  A : Inport
  B : Inport  Port=2
  C : Inport  Port=3
  Combinatorial Logic1 : CombinatorialLogic  TruthTable=[0 0;1 0 ;1 0;0 1;1 0;0 1;0 1;1 1]
  Data Type Conversion : DataTypeConversion  OutDataTypeStr=boolean
  Data Type Conversion1 : DataTypeConversion  OutDataTypeStr=double
  Demux : Demux  Outputs=2
  Mux : Mux  Inputs=3
  Carry : Outport
  Sum : Outport  Port=2
  wires:
  Demux/1 -> Sum/1
  Demux/2 -> Carry/1
  Combinatorial Logic1/1 -> Data Type Conversion1/1
  Mux/1 -> Data Type Conversion/1
  A/1 -> Mux/3
  B/1 -> Mux/2
  C/1 -> Mux/1
  Data Type Conversion1/1 -> Demux/1
  Data Type Conversion/1 -> Combinatorial Logic1/1

== system pipeline_12bit_not_ideal/pipeline_12_bit/stage_1p5_bit1/Comparator 1 ==
  Vin : Inport
  Vref : Inport  Port=2
  Output 1 or 0 : Relay  OnSwitchValue=0  OffSwitchValue=0
  Sum : Sum  Inputs=|+-
  Out : Outport
  wires:
  Sum/1 -> Output 1 or 0/1
  Vin/1 -> Sum/1
  Output 1 or 0/1 -> Out/1
  Vref/1 -> Sum/2

== system pipeline_12bit_not_ideal/pipeline_12_bit/stage_1p5_bit1/Comparator 2 ==
  Vin : Inport
  Vref : Inport  Port=2
  Output 1 or 0 : Relay  OnSwitchValue=0  OffSwitchValue=0
  Sum : Sum  Inputs=|+-
  Out : Outport
  wires:
  Sum/1 -> Output 1 or 0/1
  Vin/1 -> Sum/1
  Output 1 or 0/1 -> Out/1
  Vref/1 -> Sum/2

== system pipeline_12bit_not_ideal/pipeline_12_bit/stage_1p5_bit1/Encoder ==
  b1 : Inport
  b2 : Inport  Port=2
  " " : DataTypeConversion  OutDataTypeStr=double
  NOR : Logic  Operator=NOR  AllPortsSameDT=off  OutDataTypeStr=boolean
  NOT : Logic  Operator=NOT  AllPortsSameDT=off  OutDataTypeStr=boolean
  D0 : Outport
  D1 : Outport  Port=2
  wires:
  b2/1 -> D1/1, NOR/2
  NOR/1 -> " "/1
  " "/1 -> D0/1
  NOT/1 -> NOR/1
  b1/1 -> NOT/1

== system pipeline_12bit_not_ideal/pipeline_12_bit/stage_1p5_bit1/S//H ==
  Vin : Inport
  Clock Jitter1 : SDtoolbox/Sampling Jitter  Ts=ts  delta=delta  seed=(sum(clock))^3.33
      settings: SourceProductName=SDtoolbox
  Gain : Gain
  Saturation : Saturate  UpperLimit=1  LowerLimit=-1
  Zero-Order Hold : ZeroOrderHold  SampleTime=-1
  Out1 : Outport
  wires:
  Clock Jitter1/1 -> Gain/1  "jitter"
  Vin/1 -> Clock Jitter1/1  "original"
  Saturation/1 -> Zero-Order Hold/1
  Zero-Order Hold/1 -> Out1/1
  Gain/1 -> Saturation/1

== system pipeline_12bit_not_ideal/pipeline_12_bit/stage_1p5_bit1/Sub DAC ==
  b1 : Inport
  b2 : Inport  Port=2
  NOT : Logic  Operator=NOT  AllPortsSameDT=off  OutDataTypeStr=boolean
  Subtract : Sum  Inputs=-+
  Vdac : Outport
  wires:
  b2/1 -> Subtract/2
  b1/1 -> NOT/1
  Subtract/1 -> Vdac/1
  NOT/1 -> Subtract/1

== system pipeline_12bit_not_ideal/pipeline_12_bit/stage_1p5_bit2/Comparator 1 ==
  Vin : Inport
  Vref : Inport  Port=2
  Output 1 or 0 : Relay  OnSwitchValue=0  OffSwitchValue=0
  Sum : Sum  Inputs=|+-
  Out : Outport
  wires:
  Sum/1 -> Output 1 or 0/1
  Vin/1 -> Sum/1
  Output 1 or 0/1 -> Out/1
  Vref/1 -> Sum/2

== system pipeline_12bit_not_ideal/pipeline_12_bit/stage_1p5_bit2/Comparator 2 ==
  Vin : Inport
  Vref : Inport  Port=2
  Output 1 or 0 : Relay  OnSwitchValue=0  OffSwitchValue=0
  Sum : Sum  Inputs=|+-
  Out : Outport
  wires:
  Sum/1 -> Output 1 or 0/1
  Vin/1 -> Sum/1
  Output 1 or 0/1 -> Out/1
  Vref/1 -> Sum/2

== system pipeline_12bit_not_ideal/pipeline_12_bit/stage_1p5_bit2/Encoder ==
  b1 : Inport
  b2 : Inport  Port=2
  " " : DataTypeConversion  OutDataTypeStr=double
  NOR : Logic  Operator=NOR  AllPortsSameDT=off  OutDataTypeStr=boolean
  NOT : Logic  Operator=NOT  AllPortsSameDT=off  OutDataTypeStr=boolean
  D0 : Outport
  D1 : Outport  Port=2
  wires:
  b2/1 -> D1/1, NOR/2
  NOR/1 -> " "/1
  " "/1 -> D0/1
  NOT/1 -> NOR/1
  b1/1 -> NOT/1

== system pipeline_12bit_not_ideal/pipeline_12_bit/stage_1p5_bit2/S//H ==
  Vin : Inport
  Clock Jitter1 : SDtoolbox/Sampling Jitter  Ts=ts  delta=delta  seed=(sum(clock))^3.33
      settings: SourceProductName=SDtoolbox
  Gain : Gain
  Saturation : Saturate  UpperLimit=1  LowerLimit=-1
  Zero-Order Hold : ZeroOrderHold  SampleTime=-1
  Out1 : Outport
  wires:
  Clock Jitter1/1 -> Gain/1  "jitter"
  Vin/1 -> Clock Jitter1/1  "original"
  Saturation/1 -> Zero-Order Hold/1
  Zero-Order Hold/1 -> Out1/1
  Gain/1 -> Saturation/1

== system pipeline_12bit_not_ideal/pipeline_12_bit/stage_1p5_bit2/Sub DAC ==
  b1 : Inport
  b2 : Inport  Port=2
  NOT : Logic  Operator=NOT  AllPortsSameDT=off  OutDataTypeStr=boolean
  Subtract : Sum  Inputs=-+
  Vdac : Outport
  wires:
  b2/1 -> Subtract/2
  b1/1 -> NOT/1
  Subtract/1 -> Vdac/1
  NOT/1 -> Subtract/1

== system pipeline_12bit_not_ideal/pipeline_12_bit/stage_1p5_bit3/Comparator 1 ==
  Vin : Inport
  Vref : Inport  Port=2
  Output 1 or 0 : Relay  OnSwitchValue=0  OffSwitchValue=0
  Sum : Sum  Inputs=|+-
  Out : Outport
  wires:
  Sum/1 -> Output 1 or 0/1
  Vin/1 -> Sum/1
  Output 1 or 0/1 -> Out/1
  Vref/1 -> Sum/2

== system pipeline_12bit_not_ideal/pipeline_12_bit/stage_1p5_bit3/Comparator 2 ==
  Vin : Inport
  Vref : Inport  Port=2
  Output 1 or 0 : Relay  OnSwitchValue=0  OffSwitchValue=0
  Sum : Sum  Inputs=|+-
  Out : Outport
  wires:
  Sum/1 -> Output 1 or 0/1
  Vin/1 -> Sum/1
  Output 1 or 0/1 -> Out/1
  Vref/1 -> Sum/2

== system pipeline_12bit_not_ideal/pipeline_12_bit/stage_1p5_bit3/Encoder ==
  b1 : Inport
  b2 : Inport  Port=2
  " " : DataTypeConversion  OutDataTypeStr=double
  NOR : Logic  Operator=NOR  AllPortsSameDT=off  OutDataTypeStr=boolean
  NOT : Logic  Operator=NOT  AllPortsSameDT=off  OutDataTypeStr=boolean
  D0 : Outport
  D1 : Outport  Port=2
  wires:
  b2/1 -> D1/1, NOR/2
  NOR/1 -> " "/1
  " "/1 -> D0/1
  NOT/1 -> NOR/1
  b1/1 -> NOT/1

== system pipeline_12bit_not_ideal/pipeline_12_bit/stage_1p5_bit3/S//H ==
  Vin : Inport
  Clock Jitter1 : SDtoolbox/Sampling Jitter  Ts=ts  delta=delta  seed=(sum(clock))^3.33
      settings: SourceProductName=SDtoolbox
  Gain : Gain
  Saturation : Saturate  UpperLimit=1  LowerLimit=-1
  Zero-Order Hold : ZeroOrderHold  SampleTime=-1
  Out1 : Outport
  wires:
  Clock Jitter1/1 -> Gain/1  "jitter"
  Vin/1 -> Clock Jitter1/1  "original"
  Saturation/1 -> Zero-Order Hold/1
  Zero-Order Hold/1 -> Out1/1
  Gain/1 -> Saturation/1

== system pipeline_12bit_not_ideal/pipeline_12_bit/stage_1p5_bit3/Sub DAC ==
  b1 : Inport
  b2 : Inport  Port=2
  NOT : Logic  Operator=NOT  AllPortsSameDT=off  OutDataTypeStr=boolean
  Subtract : Sum  Inputs=-+
  Vdac : Outport
  wires:
  b2/1 -> Subtract/2
  b1/1 -> NOT/1
  Subtract/1 -> Vdac/1
  NOT/1 -> Subtract/1

== system pipeline_12bit_not_ideal/pipeline_12_bit/stage_1p5_bit4/Comparator 1 ==
  Vin : Inport
  Vref : Inport  Port=2
  Output 1 or 0 : Relay  OnSwitchValue=0  OffSwitchValue=0
  Sum : Sum  Inputs=|+-
  Out : Outport
  wires:
  Sum/1 -> Output 1 or 0/1
  Vin/1 -> Sum/1
  Output 1 or 0/1 -> Out/1
  Vref/1 -> Sum/2

== system pipeline_12bit_not_ideal/pipeline_12_bit/stage_1p5_bit4/Comparator 2 ==
  Vin : Inport
  Vref : Inport  Port=2
  Output 1 or 0 : Relay  OnSwitchValue=0  OffSwitchValue=0
  Sum : Sum  Inputs=|+-
  Out : Outport
  wires:
  Sum/1 -> Output 1 or 0/1
  Vin/1 -> Sum/1
  Output 1 or 0/1 -> Out/1
  Vref/1 -> Sum/2

== system pipeline_12bit_not_ideal/pipeline_12_bit/stage_1p5_bit4/Encoder ==
  b1 : Inport
  b2 : Inport  Port=2
  " " : DataTypeConversion  OutDataTypeStr=double
  NOR : Logic  Operator=NOR  AllPortsSameDT=off  OutDataTypeStr=boolean
  NOT : Logic  Operator=NOT  AllPortsSameDT=off  OutDataTypeStr=boolean
  D0 : Outport
  D1 : Outport  Port=2
  wires:
  b2/1 -> D1/1, NOR/2
  NOR/1 -> " "/1
  " "/1 -> D0/1
  NOT/1 -> NOR/1
  b1/1 -> NOT/1

== system pipeline_12bit_not_ideal/pipeline_12_bit/stage_1p5_bit4/S//H ==
  Vin : Inport
  Clock Jitter1 : SDtoolbox/Sampling Jitter  Ts=ts  delta=delta  seed=(sum(clock))^3.33
      settings: SourceProductName=SDtoolbox
  Gain : Gain
  Saturation : Saturate  UpperLimit=1  LowerLimit=-1
  Zero-Order Hold : ZeroOrderHold  SampleTime=-1
  Out1 : Outport
  wires:
  Clock Jitter1/1 -> Gain/1  "jitter"
  Vin/1 -> Clock Jitter1/1  "original"
  Saturation/1 -> Zero-Order Hold/1
  Zero-Order Hold/1 -> Out1/1
  Gain/1 -> Saturation/1

== system pipeline_12bit_not_ideal/pipeline_12_bit/stage_1p5_bit4/Sub DAC ==
  b1 : Inport
  b2 : Inport  Port=2
  NOT : Logic  Operator=NOT  AllPortsSameDT=off  OutDataTypeStr=boolean
  Subtract : Sum  Inputs=-+
  Vdac : Outport
  wires:
  b2/1 -> Subtract/2
  b1/1 -> NOT/1
  Subtract/1 -> Vdac/1
  NOT/1 -> Subtract/1

== system pipeline_12bit_not_ideal/pipeline_12_bit/stage_1p5_bit5/Comparator 1 ==
  Vin : Inport
  Vref : Inport  Port=2
  Output 1 or 0 : Relay  OnSwitchValue=0  OffSwitchValue=0
  Sum : Sum  Inputs=|+-
  Out : Outport
  wires:
  Sum/1 -> Output 1 or 0/1
  Vin/1 -> Sum/1
  Output 1 or 0/1 -> Out/1
  Vref/1 -> Sum/2

== system pipeline_12bit_not_ideal/pipeline_12_bit/stage_1p5_bit5/Comparator 2 ==
  Vin : Inport
  Vref : Inport  Port=2
  Output 1 or 0 : Relay  OnSwitchValue=0  OffSwitchValue=0
  Sum : Sum  Inputs=|+-
  Out : Outport
  wires:
  Sum/1 -> Output 1 or 0/1
  Vin/1 -> Sum/1
  Output 1 or 0/1 -> Out/1
  Vref/1 -> Sum/2

== system pipeline_12bit_not_ideal/pipeline_12_bit/stage_1p5_bit5/Encoder ==
  b1 : Inport
  b2 : Inport  Port=2
  " " : DataTypeConversion  OutDataTypeStr=double
  NOR : Logic  Operator=NOR  AllPortsSameDT=off  OutDataTypeStr=boolean
  NOT : Logic  Operator=NOT  AllPortsSameDT=off  OutDataTypeStr=boolean
  D0 : Outport
  D1 : Outport  Port=2
  wires:
  b2/1 -> D1/1, NOR/2
  NOR/1 -> " "/1
  " "/1 -> D0/1
  NOT/1 -> NOR/1
  b1/1 -> NOT/1

== system pipeline_12bit_not_ideal/pipeline_12_bit/stage_1p5_bit5/S//H ==
  Vin : Inport
  Clock Jitter1 : SDtoolbox/Sampling Jitter  Ts=ts  delta=delta  seed=(sum(clock))^3.33
      settings: SourceProductName=SDtoolbox
  Gain : Gain
  Saturation : Saturate  UpperLimit=1  LowerLimit=-1
  Zero-Order Hold : ZeroOrderHold  SampleTime=-1
  Out1 : Outport
  wires:
  Clock Jitter1/1 -> Gain/1  "jitter"
  Vin/1 -> Clock Jitter1/1  "original"
  Saturation/1 -> Zero-Order Hold/1
  Zero-Order Hold/1 -> Out1/1
  Gain/1 -> Saturation/1

== system pipeline_12bit_not_ideal/pipeline_12_bit/stage_1p5_bit5/Sub DAC ==
  b1 : Inport
  b2 : Inport  Port=2
  NOT : Logic  Operator=NOT  AllPortsSameDT=off  OutDataTypeStr=boolean
  Subtract : Sum  Inputs=-+
  Vdac : Outport
  wires:
  b2/1 -> Subtract/2
  b1/1 -> NOT/1
  Subtract/1 -> Vdac/1
  NOT/1 -> Subtract/1

== system pipeline_12bit_not_ideal/pipeline_12_bit/stage_1p5_bit6/Comparator 1 ==
  Vin : Inport
  Vref : Inport  Port=2
  Output 1 or 0 : Relay  OnSwitchValue=0  OffSwitchValue=0
  Sum : Sum  Inputs=|+-
  Out : Outport
  wires:
  Sum/1 -> Output 1 or 0/1
  Vin/1 -> Sum/1
  Output 1 or 0/1 -> Out/1
  Vref/1 -> Sum/2

== system pipeline_12bit_not_ideal/pipeline_12_bit/stage_1p5_bit6/Comparator 2 ==
  Vin : Inport
  Vref : Inport  Port=2
  Output 1 or 0 : Relay  OnSwitchValue=0  OffSwitchValue=0
  Sum : Sum  Inputs=|+-
  Out : Outport
  wires:
  Sum/1 -> Output 1 or 0/1
  Vin/1 -> Sum/1
  Output 1 or 0/1 -> Out/1
  Vref/1 -> Sum/2

== system pipeline_12bit_not_ideal/pipeline_12_bit/stage_1p5_bit6/Encoder ==
  b1 : Inport
  b2 : Inport  Port=2
  " " : DataTypeConversion  OutDataTypeStr=double
  NOR : Logic  Operator=NOR  AllPortsSameDT=off  OutDataTypeStr=boolean
  NOT : Logic  Operator=NOT  AllPortsSameDT=off  OutDataTypeStr=boolean
  D0 : Outport
  D1 : Outport  Port=2
  wires:
  b2/1 -> D1/1, NOR/2
  NOR/1 -> " "/1
  " "/1 -> D0/1
  NOT/1 -> NOR/1
  b1/1 -> NOT/1

== system pipeline_12bit_not_ideal/pipeline_12_bit/stage_1p5_bit6/S//H ==
  Vin : Inport
  Clock Jitter1 : SDtoolbox/Sampling Jitter  Ts=ts  delta=delta  seed=(sum(clock))^3.33
      settings: SourceProductName=SDtoolbox
  Gain : Gain
  Saturation : Saturate  UpperLimit=1  LowerLimit=-1
  Zero-Order Hold : ZeroOrderHold  SampleTime=-1
  Out1 : Outport
  wires:
  Clock Jitter1/1 -> Gain/1  "jitter"
  Vin/1 -> Clock Jitter1/1  "original"
  Saturation/1 -> Zero-Order Hold/1
  Zero-Order Hold/1 -> Out1/1
  Gain/1 -> Saturation/1

== system pipeline_12bit_not_ideal/pipeline_12_bit/stage_1p5_bit6/Sub DAC ==
  b1 : Inport
  b2 : Inport  Port=2
  NOT : Logic  Operator=NOT  AllPortsSameDT=off  OutDataTypeStr=boolean
  Subtract : Sum  Inputs=-+
  Vdac : Outport
  wires:
  b2/1 -> Subtract/2
  b1/1 -> NOT/1
  Subtract/1 -> Vdac/1
  NOT/1 -> Subtract/1

== system pipeline_12bit_not_ideal/pipeline_12_bit/stage_1p5_bit7/Comparator 1 ==
  Vin : Inport
  Vref : Inport  Port=2
  Output 1 or 0 : Relay  OnSwitchValue=0  OffSwitchValue=0
  Sum : Sum  Inputs=|+-
  Out : Outport
  wires:
  Sum/1 -> Output 1 or 0/1
  Vin/1 -> Sum/1
  Output 1 or 0/1 -> Out/1
  Vref/1 -> Sum/2

== system pipeline_12bit_not_ideal/pipeline_12_bit/stage_1p5_bit7/Comparator 2 ==
  Vin : Inport
  Vref : Inport  Port=2
  Output 1 or 0 : Relay  OnSwitchValue=0  OffSwitchValue=0
  Sum : Sum  Inputs=|+-
  Out : Outport
  wires:
  Sum/1 -> Output 1 or 0/1
  Vin/1 -> Sum/1
  Output 1 or 0/1 -> Out/1
  Vref/1 -> Sum/2

== system pipeline_12bit_not_ideal/pipeline_12_bit/stage_1p5_bit7/Encoder ==
  b1 : Inport
  b2 : Inport  Port=2
  " " : DataTypeConversion  OutDataTypeStr=double
  NOR : Logic  Operator=NOR  AllPortsSameDT=off  OutDataTypeStr=boolean
  NOT : Logic  Operator=NOT  AllPortsSameDT=off  OutDataTypeStr=boolean
  D0 : Outport
  D1 : Outport  Port=2
  wires:
  b2/1 -> D1/1, NOR/2
  NOR/1 -> " "/1
  " "/1 -> D0/1
  NOT/1 -> NOR/1
  b1/1 -> NOT/1

== system pipeline_12bit_not_ideal/pipeline_12_bit/stage_1p5_bit7/S//H ==
  Vin : Inport
  Clock Jitter1 : SDtoolbox/Sampling Jitter  Ts=ts  delta=delta  seed=(sum(clock))^3.33
      settings: SourceProductName=SDtoolbox
  Gain : Gain
  Saturation : Saturate  UpperLimit=1  LowerLimit=-1
  Zero-Order Hold : ZeroOrderHold  SampleTime=-1
  Out1 : Outport
  wires:
  Clock Jitter1/1 -> Gain/1  "jitter"
  Vin/1 -> Clock Jitter1/1  "original"
  Saturation/1 -> Zero-Order Hold/1
  Zero-Order Hold/1 -> Out1/1
  Gain/1 -> Saturation/1

== system pipeline_12bit_not_ideal/pipeline_12_bit/stage_1p5_bit7/Sub DAC ==
  b1 : Inport
  b2 : Inport  Port=2
  NOT : Logic  Operator=NOT  AllPortsSameDT=off  OutDataTypeStr=boolean
  Subtract : Sum  Inputs=-+
  Vdac : Outport
  wires:
  b2/1 -> Subtract/2
  b1/1 -> NOT/1
  Subtract/1 -> Vdac/1
  NOT/1 -> Subtract/1

== system pipeline_12bit_not_ideal/pipeline_12_bit/stage_2p5_bit/Comparator 1 ==
  Vin : Inport
  Vref : Inport  Port=2
  Output 1 or 0 : Relay  OnSwitchValue=0  OffSwitchValue=0
  Sum : Sum  Inputs=|+-
  Out : Outport
  wires:
  Sum/1 -> Output 1 or 0/1
  Vin/1 -> Sum/1
  Output 1 or 0/1 -> Out/1
  Vref/1 -> Sum/2

== system pipeline_12bit_not_ideal/pipeline_12_bit/stage_2p5_bit/Comparator 2 ==
  Vin : Inport
  Vref : Inport  Port=2
  Output 1 or 0 : Relay  OnSwitchValue=0  OffSwitchValue=0
  Sum : Sum  Inputs=|+-
  Out : Outport
  wires:
  Sum/1 -> Output 1 or 0/1
  Vin/1 -> Sum/1
  Output 1 or 0/1 -> Out/1
  Vref/1 -> Sum/2

== system pipeline_12bit_not_ideal/pipeline_12_bit/stage_2p5_bit/Comparator 3 ==
  Vin : Inport
  Vref : Inport  Port=2
  Output 1 or 0 : Relay  OnSwitchValue=0  OffSwitchValue=0
  Sum : Sum  Inputs=|+-
  Out : Outport
  wires:
  Sum/1 -> Output 1 or 0/1
  Vin/1 -> Sum/1
  Output 1 or 0/1 -> Out/1
  Vref/1 -> Sum/2

== system pipeline_12bit_not_ideal/pipeline_12_bit/stage_2p5_bit/Comparator 4 ==
  Vin : Inport
  Vref : Inport  Port=2
  Output 1 or 0 : Relay  OnSwitchValue=0  OffSwitchValue=0
  Sum : Sum  Inputs=|+-
  Out : Outport
  wires:
  Sum/1 -> Output 1 or 0/1
  Vin/1 -> Sum/1
  Output 1 or 0/1 -> Out/1
  Vref/1 -> Sum/2

== system pipeline_12bit_not_ideal/pipeline_12_bit/stage_2p5_bit/Comparator 5 ==
  Vin : Inport
  Vref : Inport  Port=2
  Output 1 or 0 : Relay  OnSwitchValue=0  OffSwitchValue=0
  Sum : Sum  Inputs=|+-
  Out : Outport
  wires:
  Sum/1 -> Output 1 or 0/1
  Vin/1 -> Sum/1
  Output 1 or 0/1 -> Out/1
  Vref/1 -> Sum/2

== system pipeline_12bit_not_ideal/pipeline_12_bit/stage_2p5_bit/Comparator 6 ==
  Vin : Inport
  Vref : Inport  Port=2
  Output 1 or 0 : Relay  OnSwitchValue=0  OffSwitchValue=0
  Sum : Sum  Inputs=|+-
  Out : Outport
  wires:
  Sum/1 -> Output 1 or 0/1
  Vin/1 -> Sum/1
  Output 1 or 0/1 -> Out/1
  Vref/1 -> Sum/2

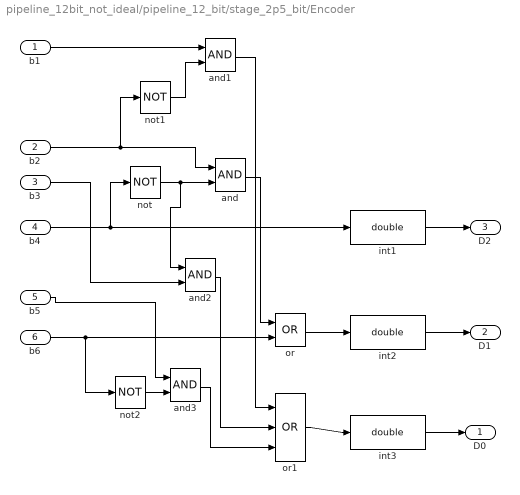
== system pipeline_12bit_not_ideal/pipeline_12_bit/stage_2p5_bit/Encoder ==
  b1 : Inport
  b2 : Inport  Port=2
  b3 : Inport  Port=3
  b4 : Inport  Port=4
  b5 : Inport  Port=5
  b6 : Inport  Port=6
  and{,1..3} (4 alike) : Logic  AllPortsSameDT=off  OutDataTypeStr=boolean
  int1 : DataTypeConversion  OutDataTypeStr=double
  int2 : DataTypeConversion  OutDataTypeStr=double
  int3 : DataTypeConversion  OutDataTypeStr=double
  not : Logic  Operator=NOT  AllPortsSameDT=off  OutDataTypeStr=boolean
  not1 : Logic  Operator=NOT  AllPortsSameDT=off  OutDataTypeStr=boolean
  not2 : Logic  Operator=NOT  AllPortsSameDT=off  OutDataTypeStr=boolean
  or : Logic  Operator=OR  AllPortsSameDT=off  OutDataTypeStr=boolean
  or1 : Logic  Operator=OR  Inputs=3  AllPortsSameDT=off  OutDataTypeStr=boolean
  D0 : Outport
  D1 : Outport  Port=2
  D2 : Outport  Port=3
  wires:
  b4/1 -> not/1, int1/1
  not/1 -> and/2, and2/1
  b2/1 -> and/1, not1/1
  b6/1 -> or/2, not2/1
  and/1 -> or/1
  or/1 -> int2/1
  or1/1 -> int3/1
  b1/1 -> and1/1
  not1/1 -> and1/2
  and1/1 -> or1/1
  b3/1 -> and2/2
  and2/1 -> or1/2
  not2/1 -> and3/2
  b5/1 -> and3/1
  int2/1 -> D1/1
  int3/1 -> D0/1
  and3/1 -> or1/3
  int1/1 -> D2/1

== system pipeline_12bit_not_ideal/pipeline_12_bit/stage_2p5_bit/S//H ==
  Vin : Inport
  Clock Jitter1 : SDtoolbox/Sampling Jitter  Ts=ts  delta=delta  seed=(sum(clock))^3.33
      settings: SourceProductName=SDtoolbox
  Gain : Gain
  Saturation : Saturate  UpperLimit=1  LowerLimit=-1
  Zero-Order Hold : ZeroOrderHold  SampleTime=-1
  Out1 : Outport
  wires:
  Clock Jitter1/1 -> Gain/1  "jitter"
  Vin/1 -> Clock Jitter1/1  "original"
  Saturation/1 -> Zero-Order Hold/1
  Zero-Order Hold/1 -> Out1/1
  Gain/1 -> Saturation/1

== system pipeline_12bit_not_ideal/pipeline_12_bit/stage_2p5_bit/Sub DAC ==
  b1 : Inport
  b2 : Inport  Port=2
  b3 : Inport  Port=3
  b4 : Inport  Port=4
  b5 : Inport  Port=5
  b6 : Inport  Port=6
  Constant : Constant  Value=6
  Gain : Gain  Gain=2
  Gain1 : Gain  Gain=0.5
  Sum : Sum  Inputs=++++++
  Sum1 : Sum  Inputs=|+-
  Vdac : Outport
  wires:
  b1/1 -> Sum/1
  b2/1 -> Sum/2
  b3/1 -> Sum/3
  b4/1 -> Sum/4
  b5/1 -> Sum/5
  b6/1 -> Sum/6
  Sum/1 -> Gain/1
  Gain/1 -> Sum1/1
  Constant/1 -> Sum1/2
  Sum1/1 -> Gain1/1
  Gain1/1 -> Vdac/1

== system pipeline_12bit_not_ideal/pipeline_12_bit/stage_3_bit_flash/Comparator 1 ==
  Vin : Inport
  Vref : Inport  Port=2
  Output 1 or 0 : Relay  OnSwitchValue=0  OffSwitchValue=0
  Sum : Sum  Inputs=|+-
  Out : Outport
  wires:
  Sum/1 -> Output 1 or 0/1
  Vin/1 -> Sum/1
  Output 1 or 0/1 -> Out/1
  Vref/1 -> Sum/2

== system pipeline_12bit_not_ideal/pipeline_12_bit/stage_3_bit_flash/Comparator 2 ==
  Vin : Inport
  Vref : Inport  Port=2
  Output 1 or 0 : Relay  OnSwitchValue=0  OffSwitchValue=0
  Sum : Sum  Inputs=|+-
  Out : Outport
  wires:
  Sum/1 -> Output 1 or 0/1
  Vin/1 -> Sum/1
  Output 1 or 0/1 -> Out/1
  Vref/1 -> Sum/2

== system pipeline_12bit_not_ideal/pipeline_12_bit/stage_3_bit_flash/Comparator 3 ==
  Vin : Inport
  Vref : Inport  Port=2
  Output 1 or 0 : Relay  OnSwitchValue=0  OffSwitchValue=0
  Sum : Sum  Inputs=|+-
  Out : Outport
  wires:
  Sum/1 -> Output 1 or 0/1
  Vin/1 -> Sum/1
  Output 1 or 0/1 -> Out/1
  Vref/1 -> Sum/2

== system pipeline_12bit_not_ideal/pipeline_12_bit/stage_3_bit_flash/Comparator 4 ==
  Vin : Inport
  Vref : Inport  Port=2
  Output 1 or 0 : Relay  OnSwitchValue=0  OffSwitchValue=0
  Sum : Sum  Inputs=|+-
  Out : Outport
  wires:
  Sum/1 -> Output 1 or 0/1
  Vin/1 -> Sum/1
  Output 1 or 0/1 -> Out/1
  Vref/1 -> Sum/2

== system pipeline_12bit_not_ideal/pipeline_12_bit/stage_3_bit_flash/Comparator 5 ==
  Vin : Inport
  Vref : Inport  Port=2
  Output 1 or 0 : Relay  OnSwitchValue=0  OffSwitchValue=0
  Sum : Sum  Inputs=|+-
  Out : Outport
  wires:
  Sum/1 -> Output 1 or 0/1
  Vin/1 -> Sum/1
  Output 1 or 0/1 -> Out/1
  Vref/1 -> Sum/2

== system pipeline_12bit_not_ideal/pipeline_12_bit/stage_3_bit_flash/Comparator 6 ==
  Vin : Inport
  Vref : Inport  Port=2
  Output 1 or 0 : Relay  OnSwitchValue=0  OffSwitchValue=0
  Sum : Sum  Inputs=|+-
  Out : Outport
  wires:
  Sum/1 -> Output 1 or 0/1
  Vin/1 -> Sum/1
  Output 1 or 0/1 -> Out/1
  Vref/1 -> Sum/2

== system pipeline_12bit_not_ideal/pipeline_12_bit/stage_3_bit_flash/Comparator 7 ==
  Vin : Inport
  Vref : Inport  Port=2
  Output 1 or 0 : Relay  OnSwitchValue=0  OffSwitchValue=0
  Sum : Sum  Inputs=|+-
  Out : Outport
  wires:
  Sum/1 -> Output 1 or 0/1
  Vin/1 -> Sum/1
  Output 1 or 0/1 -> Out/1
  Vref/1 -> Sum/2

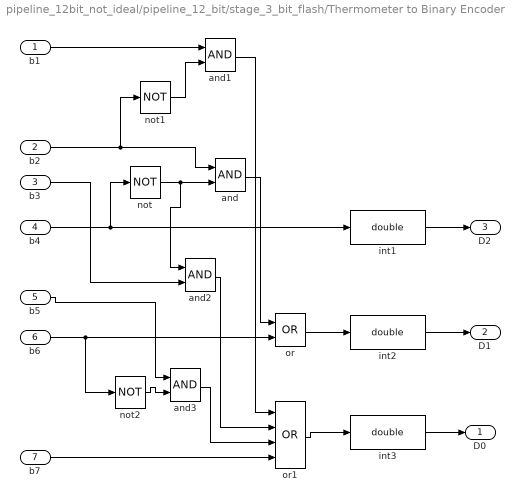
== system pipeline_12bit_not_ideal/pipeline_12_bit/stage_3_bit_flash/Thermometer to Binary Encoder ==
  b1 : Inport
  b2 : Inport  Port=2
  b3 : Inport  Port=3
  b4 : Inport  Port=4
  b5 : Inport  Port=5
  b6 : Inport  Port=6
  b7 : Inport  Port=7
  and{,1..3} (4 alike) : Logic  AllPortsSameDT=off  OutDataTypeStr=boolean
  int1 : DataTypeConversion  OutDataTypeStr=double
  int2 : DataTypeConversion  OutDataTypeStr=double
  int3 : DataTypeConversion  OutDataTypeStr=double
  not : Logic  Operator=NOT  AllPortsSameDT=off  OutDataTypeStr=boolean
  not1 : Logic  Operator=NOT  AllPortsSameDT=off  OutDataTypeStr=boolean
  not2 : Logic  Operator=NOT  AllPortsSameDT=off  OutDataTypeStr=boolean
  or : Logic  Operator=OR  AllPortsSameDT=off  OutDataTypeStr=boolean
  or1 : Logic  Operator=OR  Inputs=4  AllPortsSameDT=off  OutDataTypeStr=boolean
  D0 : Outport
  D1 : Outport  Port=2
  D2 : Outport  Port=3
  wires:
  b4/1 -> not/1, int1/1
  not/1 -> and/2, and2/1
  b2/1 -> and/1, not1/1
  b6/1 -> or/2, not2/1
  and/1 -> or/1
  or/1 -> int2/1
  or1/1 -> int3/1
  b1/1 -> and1/1
  not1/1 -> and1/2
  and1/1 -> or1/1
  b3/1 -> and2/2
  and2/1 -> or1/2
  b7/1 -> or1/4
  not2/1 -> and3/2
  b5/1 -> and3/1
  int2/1 -> D1/1
  int3/1 -> D0/1
  and3/1 -> or1/3
  int1/1 -> D2/1
